simulink model "tx80211a6s"  (R2015b)
settings: Solver=FixedStepDiscrete  SolverMode=SingleTasking  StartTime=0.0  StopTime=46*tpf  RelTol=1e-3
PreLoadFcn:
  | [stx, stb, spi, spq, ntf, cii, cpp, css] = tx80211a_r0;
InitFcn:
  | if ~exist('srx','var')
  | [stx, stb, spi, spq, ntf, cii, cpp, css] = tx80211a_r0;
  | end
  | bitrate = 6e6; % 6 Mbits per second
  | crf = 2; % constant redundancy factor (from conv enc)
  | nepsc = 16; % #empty+pilot subcarriers
  | ncps = 16; % #cyclic prefix samples
  | ndbpf = 24; % #data bits per frame
  | ncbpf = ndbpf * crf; % #coded bits per frame
  | nscpf = ncbpf + nepsc; % #subcarriers per frame
  | nspf = nscpf + 16; % #samples per frame
  | tps = 1e-6; %tpf/nspf; % sample time
  | tpf = tps*nspf; %ndbpf/bitrate; % frame time
undefined symbols (not defined in the file): cpp, css, ntf, spi, spq, stb
libraries: simulink x43, hdlsllib x35, dspsigops x2, commcnvcod2 x1, dspxfrm3 x1
(part 2 of 2)

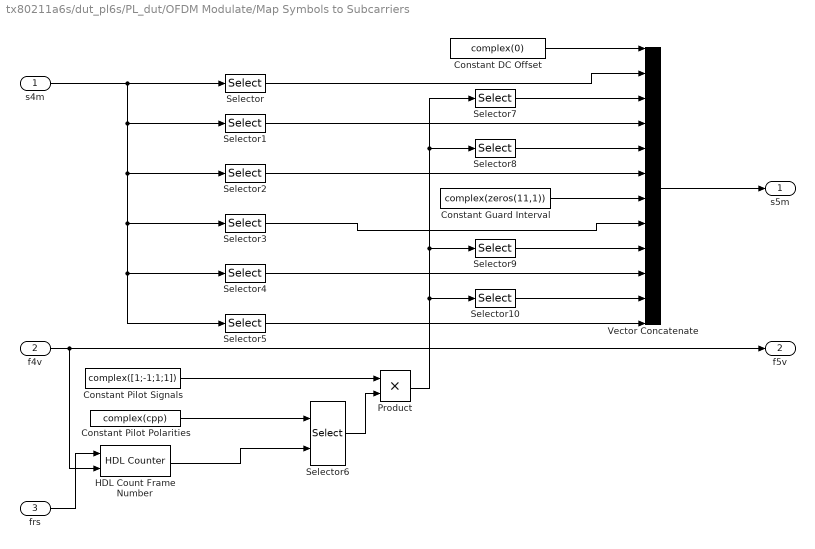
== system tx80211a6s/dut_pl6s/PL_dut/OFDM Modulate/Map Symbols to Subcarriers ==
  s4m : Inport
  f4v : Inport  Port=2
  frs : Inport  Port=3
  Constant DC Offset : Constant  Value=complex(0)  OutDataTypeStr=fixdt(1,16,14)  SampleTime=tps
  Constant Guard Interval : Constant  Value=complex(zeros(11,1))  OutDataTypeStr=fixdt(1,16,14)  SampleTime=tps
  Constant Pilot Polarities : Constant  Value=complex(cpp)  OutDataTypeStr=fixdt(1,16,14)  SampleTime=tps
  Constant Pilot Signals : Constant  Value=complex([1;-1;1;1])  OutDataTypeStr=fixdt(1,16,14)  SampleTime=tps
  HDL Count Frame Number : hdlsllib/HDL Operations/HDL Counter  CountType=Count limited  CountInit=0  CountStep=1  CountMax=127  CountFromType=Initial value  CountFrom=0  CountResetPort=on  CountLoadPort=off  CountEnbPort=on  CountDirPort=off  CountDataType=Unsigned  CountWordLen=8  CountFracLen=0  CountSampTime=1
  Product : Product  OutDataTypeStr=fixdt(1,16,14)
  Selector : Selector  IndexMode=Zero-based  InputPortWidth=48  IndexOptions=Index vector (dialog)  Indices=24:29  OutputSizes=1
  Selector1 : Selector  IndexMode=Zero-based  InputPortWidth=48  IndexOptions=Index vector (dialog)  Indices=30:42  OutputSizes=1
  Selector10 : Selector  IndexMode=Zero-based  InputPortWidth=4  IndexOptions=Index vector (dialog)  Indices=3  OutputSizes=1
  Selector2 : Selector  IndexMode=Zero-based  InputPortWidth=48  IndexOptions=Index vector (dialog)  Indices=43:47  OutputSizes=1
  Selector3 : Selector  IndexMode=Zero-based  InputPortWidth=48  IndexOptions=Index vector (dialog)  Indices=0:4  OutputSizes=1
  Selector4 : Selector  IndexMode=Zero-based  InputPortWidth=48  IndexOptions=Index vector (dialog)  Indices=5:17  OutputSizes=1
  Selector5 : Selector  IndexMode=Zero-based  InputPortWidth=48  IndexOptions=Index vector (dialog)  Indices=18:23  OutputSizes=1
  Selector6 : Selector  IndexMode=Zero-based  InputPortWidth=127  IndexOptions=Starting index (port)  Indices=[1 3]  OutputSizes=1
  Selector7 : Selector  IndexMode=Zero-based  InputPortWidth=4  IndexOptions=Index vector (dialog)  Indices=0  OutputSizes=1
  Selector8 : Selector  IndexMode=Zero-based  InputPortWidth=4  IndexOptions=Index vector (dialog)  Indices=1  OutputSizes=1
  Selector9 : Selector  IndexMode=Zero-based  InputPortWidth=4  IndexOptions=Index vector (dialog)  Indices=2  OutputSizes=1
  Vector Concatenate : Concatenate  NumInputs=12
  s5m : Outport
  f5v : Outport  Port=2
  wires:
  s4m/1 -> Selector2/1, Selector3/1, Selector4/1, Selector5/1, Selector1/1, Selector/1
  frs/1 -> HDL Count Frame Number/1
  Constant Pilot Polarities/1 -> Selector6/1
  Constant Pilot Signals/1 -> Product/1
  Selector6/1 -> Product/2
  Selector/1 -> Vector Concatenate/2
  Selector1/1 -> Vector Concatenate/4
  Selector2/1 -> Vector Concatenate/6
  Selector3/1 -> Vector Concatenate/8
  Selector4/1 -> Vector Concatenate/10
  Selector5/1 -> Vector Concatenate/12
  Constant DC Offset/1 -> Vector Concatenate/1
  Selector10/1 -> Vector Concatenate/11
  Selector9/1 -> Vector Concatenate/9
  Selector8/1 -> Vector Concatenate/5
  Selector7/1 -> Vector Concatenate/3
  Constant Guard Interval/1 -> Vector Concatenate/7
  Vector Concatenate/1 -> s5m/1
  Product/1 -> Selector10/1, Selector9/1, Selector8/1, Selector7/1
  f4v/1 -> HDL Count Frame Number/2, f5v/1
  HDL Count Frame Number/1 -> Selector6/2

== system tx80211a6s/dut_pl6s/PL_dut/OFDM Modulate/Prepend Cyclic Prefix ==
  s7s : Inport
  f7v : Inport  Port=2
  frs : Inport  Port=3
  Delay1 : Delay  DelayLength=64  ExternalReset=Level  SampleTime=tps
      settings: InputPortMap=u0,r5
  Delay2 : Delay  DelayLength=48  ExternalReset=Level  SampleTime=tps
      settings: InputPortMap=u0,r5
  Delay3 : Delay  DelayLength=64  ExternalReset=Level  SampleTime=tps
      settings: InputPortMap=u0,r5
  Logical OR : Logic  Operator=OR  IconShape=distinctive  AllPortsSameDT=off  OutDataTypeStr=boolean
  Switch : Switch  Criteria=u2 ~= 0
  s8s : Outport
  f8v : Outport  Port=2
  wires:
  Switch/1 -> s8s/1
  s7s/1 -> Switch/3, Delay1/1
  Delay2/1 -> Logical OR/1
  Delay1/1 -> Switch/1
  frs/1 -> Delay2/2, Delay1/2, Delay3/2
  Logical OR/1 -> f8v/1
  Delay3/1 -> Switch/2, Logical OR/2
  f7v/1 -> Delay3/1, Delay2/1
